simulink model "testModel_Rx16Tx32_regs"  (R2021b)
settings: Solver=FixedStepDiscrete  StartTime=0.0  StopTime=10.0  RelTol=1e-3
libraries: simulink x1
settings Model: DataTypeOverride=Off  Creator=tcollins  LastModifiedBy=tcollins
settings SolverCC: AlgebraicLoopSolver=TrustRegion
settings DataIOCC: LimitDataPoints=on  SaveOutput=off  SaveTime=off  ReturnWorkspaceOutputs=off
settings OptimizationCC: BlockReduction=off  ConditionallyExecuteInputs=off  DefaultParameterBehavior=Inlined  LifeSpan=inf
settings DebuggingCC: AlgebraicLoopMsg=error  SingleTaskRateTransMsg=error  AllowSymbolicDim=off  StrictBusMsg=ErrorOnBusTreatedAsVector  SFUnexpectedBacktrackingDiag=warning  SFNoUnconditionalDefaultTransitionDiag=warning  SFExecutionAtInitializationDiag=none  SFMachineParentedDataDiag=warning  ArithmeticOperatorsInVariantConditions=warning
settings HardwareCC: ProdBitPerPointer=32  ProdBitPerSizeT=32  ProdBitPerPtrDiffT=32  ProdLargestAtomicFloat=None  ProdIntDivRoundTo=Undefined  ProdEndianess=Unspecified  ProdWordSize=32  ProdHWDeviceType=ASIC/FPGA->ASIC/FPGA  ProdEqTarget=off
settings SFSimCC: SimUseLocalCustomCode=off  CustomCodeUndefinedFunction=UseInterfaceOnly
settings RTWCC: RTWUseLocalCustomCode=off
settings CodeAppCC: StateflowObjectComments=on
settings GRTTargetCC: TargetLangStandard=C89/C90 (ANSI)
settings ConfigComp: CovScope=ReferencedModels  CovMetricSettings=dw  CovSaveCumulativeToWorkspaceVar=on  CovSaveSingleToWorkspaceVar=on  CovExternalEMLEnable=off  CovSFcnEnable=off

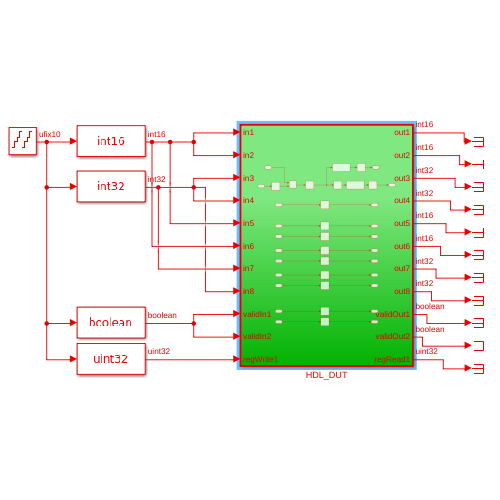
[thumbnail: Simulink's stored preview of the top-level diagram]
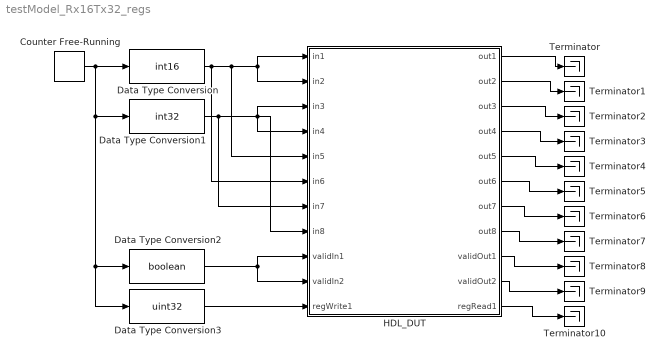
== system testModel_Rx16Tx32_regs ==
  Counter Free-Running : simulink/Sources/Counter Free-Running  NumBits=10  tsamp=1
  Data Type Conversion : DataTypeConversion  OutDataTypeStr=int16
  Data Type Conversion1 : DataTypeConversion  OutDataTypeStr=int32
  Data Type Conversion2 : DataTypeConversion  OutDataTypeStr=boolean
  Data Type Conversion3 : DataTypeConversion  OutDataTypeStr=uint32
  HDL_DUT : Subsystem  TreatAsAtomicUnit=on
  Terminator{,1..10} (11 alike) : Terminator
  wires:
  HDL_DUT/1(out1) -> Terminator/1
  HDL_DUT/2(out2) -> Terminator1/1
  HDL_DUT/3(out3) -> Terminator2/1
  HDL_DUT/4(out4) -> Terminator3/1
  Data Type Conversion/1 -> HDL_DUT/2(in2), HDL_DUT/1(in1), HDL_DUT/5(in5), HDL_DUT/6(in6)
  HDL_DUT/5(out5) -> Terminator4/1
  HDL_DUT/6(out6) -> Terminator5/1
  HDL_DUT/7(out7) -> Terminator6/1
  HDL_DUT/8(out8) -> Terminator7/1
  Data Type Conversion1/1 -> HDL_DUT/4(in4), HDL_DUT/3(in3), HDL_DUT/8(in8), HDL_DUT/7(in7)
  Data Type Conversion2/1 -> HDL_DUT/10(validIn2), HDL_DUT/9(validIn1)
  HDL_DUT/9(validOut1) -> Terminator8/1
  HDL_DUT/10(validOut2) -> Terminator9/1
  Counter Free-Running/1 -> Data Type Conversion3/1, Data Type Conversion2/1, Data Type Conversion1/1, Data Type Conversion/1
  Data Type Conversion3/1 -> HDL_DUT/11(regWrite1)
  HDL_DUT/11(regRead1) -> Terminator10/1

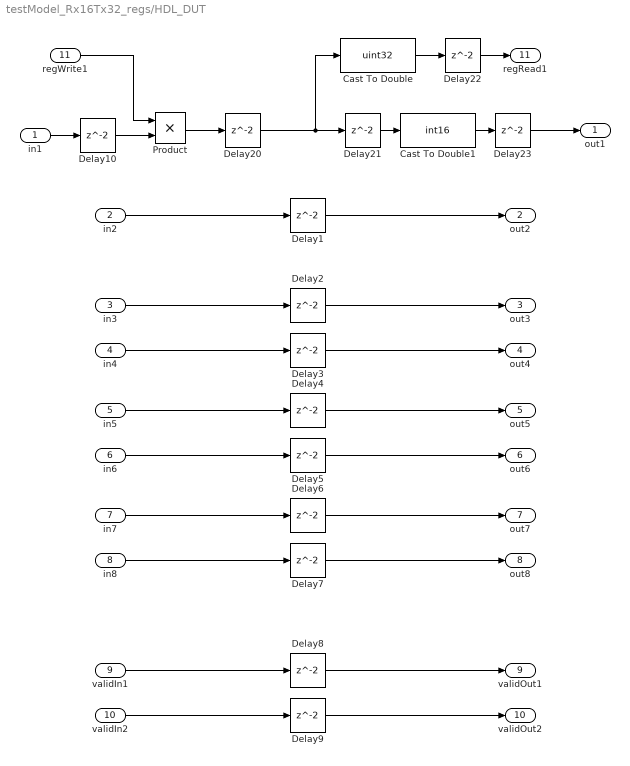
== system testModel_Rx16Tx32_regs/HDL_DUT ==
  in1 : Inport
  in2 : Inport  Port=2
  in3 : Inport  Port=3
  in4 : Inport  Port=4
  in5 : Inport  Port=5
  in6 : Inport  Port=6
  in7 : Inport  Port=7
  in8 : Inport  Port=8
  validIn1 : Inport  Port=9
  validIn2 : Inport  Port=10
  regWrite1 : Inport  Port=11
  Cast To Double : DataTypeConversion  OutDataTypeStr=uint32
  Cast To Double1 : DataTypeConversion  OutDataTypeStr=int16
  Delay{1..10,20..23} (14 alike) : Delay
  Product : Product
  out1 : Outport  VectorParamsAs1DForOutWhenUnconnected=off
  out2 : Outport  Port=2  VectorParamsAs1DForOutWhenUnconnected=off
  out3 : Outport  Port=3  VectorParamsAs1DForOutWhenUnconnected=off
  out4 : Outport  Port=4  VectorParamsAs1DForOutWhenUnconnected=off
  out5 : Outport  Port=5  VectorParamsAs1DForOutWhenUnconnected=off
  out6 : Outport  Port=6  VectorParamsAs1DForOutWhenUnconnected=off
  out7 : Outport  Port=7  VectorParamsAs1DForOutWhenUnconnected=off
  out8 : Outport  Port=8  VectorParamsAs1DForOutWhenUnconnected=off
  validOut1 : Outport  Port=9  VectorParamsAs1DForOutWhenUnconnected=off
  validOut2 : Outport  Port=10  VectorParamsAs1DForOutWhenUnconnected=off
  regRead1 : Outport  Port=11  VectorParamsAs1DForOutWhenUnconnected=off
  wires:
  Delay1/1 -> out2/1
  in2/1 -> Delay1/1
  Delay3/1 -> out4/1
  in3/1 -> Delay2/1
  in4/1 -> Delay3/1
  Delay2/1 -> out3/1
  Delay6/1 -> out7/1
  Delay5/1 -> out6/1
  in7/1 -> Delay6/1
  in8/1 -> Delay7/1
  in5/1 -> Delay4/1
  in6/1 -> Delay5/1
  Delay4/1 -> out5/1
  Delay7/1 -> out8/1
  Delay8/1 -> validOut1/1
  validIn1/1 -> Delay8/1
  validIn2/1 -> Delay9/1
  Delay9/1 -> validOut2/1
  Delay10/1 -> Product/2
  Delay20/1 -> Cast To Double/1, Delay21/1
  in1/1 -> Delay10/1
  Delay21/1 -> Cast To Double1/1
  Cast To Double/1 -> Delay22/1
  Delay23/1 -> out1/1
  Product/1 -> Delay20/1
  regWrite1/1 -> Product/1
  Cast To Double1/1 -> Delay23/1
  Delay22/1 -> regRead1/1
